simulink model "triggered_counter_blk"  (R2019a)
settings: Solver=VariableStepAuto  StartTime=0.0  StopTime=10.0  RelTol=1e-3
libraries: xbsIndex_r4 x5
settings Model: Creator=mybur  LastModifiedBy=mybur

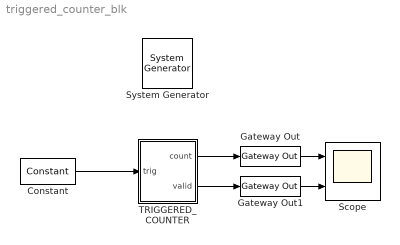
== system triggered_counter_blk ==
  " System Generator" : xbsIndex_r4/ System Generator  Tag=genX  xilinxfamily=kintex7  part=xc7k325t  speed=-3  package=fbg676  synthesis_tool=Vivado  clock_wrapper=Clock Enables  directory=./netlist  proj_type=Vivado  Synth_file=Vivado Synthesis Defaults  Impl_file=Vivado Implementation Defaults  testbench=off  simulink_period=1  sysclk_period=10  dcm_input_clock_period=10  incr_netlist=off  trim_vbits=Everywhere in SubSystem  dbl_ovrd=According to Block Masks  core_generation=According to Block Masks  run_coregen=off  deprecated_control=off  eval_field=0  block_type=sysgen
  Constant : xbsIndex_r4/Constant  const=1.0  gui_display_data_type=Fixed-point  arith_type=Unsigned  n_bits=1  bin_pt=0  preci_type=Single  exp_width=8  frac_width=24  explicit_period=on  period=1  equ=P=C  opselect=C  inp2=PCIN>>17  opr=+  inp1=P  carry=CIN  dbl_ovrd=off  block_type=constant
  Gateway Out : xbsIndex_r4/Gateway Out  inherit_from_input=off  hdl_port=on  rows=1  columns=1  UseAsDAC=off  DACChannel='1'  interface=None  automatic_assignment=on  address_offset=hex2dec('00')  intf_name=''  intf_description=''  timing_constraint=None  locs_specified=off  LOCs={}  io_standard={}  block_type=gatewayout
  Gateway Out1 : xbsIndex_r4/Gateway Out  inherit_from_input=off  hdl_port=on  rows=1  columns=1  UseAsDAC=off  DACChannel='1'  interface=None  automatic_assignment=on  address_offset=hex2dec('00')  intf_name=''  intf_description=''  timing_constraint=None  locs_specified=off  LOCs={}  io_standard={}  block_type=gatewayout
  Scope : Scope  NumInputPorts=2
  TRIGGERED_COUNTER : Subsystem  mask{len=5}
      mask prompts: len "Run length"
      mask init:
      | Simulink.Block.eval([gcb, '/triggered_counter']);
  wires:
  Constant/1 -> TRIGGERED_COUNTER/1(trig)
  Gateway Out/1 -> Scope/1
  TRIGGERED_COUNTER/1(count) -> Gateway Out/1
  Gateway Out1/1 -> Scope/2
  TRIGGERED_COUNTER/2(valid) -> Gateway Out1/1

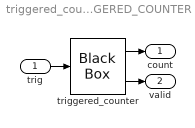
== system triggered_counter_blk/TRIGGERED_COUNTER ==
  trig : Inport
  triggered_counter : xbsIndex_r4/Black Box  init_code=triggered_counter_config  sim_method=ISE Simulator  verbose=off  block_type=blackbox2
  count : Outport
  valid : Outport  Port=2
  wires:
  trig/1 -> triggered_counter/1
  triggered_counter/1 -> count/1
  triggered_counter/2 -> valid/1
